simulink model "tx2"  (R2022a)
settings: Solver=FixedStepDiscrete  StartTime=0.0  StopTime=3.1e6  FixedStep=1  RelTol=1e-3
undefined symbols (not defined in the file or in its folder): rom_bf1, rom_bf2, rom_bf3, rom_bf4, rom_bf5, rom_bf6, rom_bf7, rom_bf8, rom_pilot_tt
libraries: hdlsllib x809, whdlutilities x460, whdlmod x104, whdledac x26, simulink x3
(part 25 of 27)

== system tx2/Subsystem4/OFDM_process1/OFDM_process1_bf1/OFDM_BF1/recover_valid_specify ==
  data_in : Inport
  start_in : Inport  Port=2  OutDataTypeStr=boolean
  end_in : Inport  Port=3  OutDataTypeStr=boolean
  Constant : Constant  Value=0  OutDataTypeStr=boolean
  Data Type Conversion1 : DataTypeConversion  OutDataTypeStr=boolean  SaturateOnIntegerOverflow=off  RndMeth=Floor
  Delay : Delay  InitialCondition=0
  Delay1 : Delay  DelayLength=1  InitialCondition=0
  Delay2 : Delay  DelayLength=1  InitialCondition=0
  Delay3 : Delay  InitialCondition=0
  HDL Counter1 : hdlsllib/Sources/HDL Counter  CountType=Count limited  CountInit=0  CountStep=1  CountMax=1  CountFromType=Initial value  CountFrom=0  CountResetPort=off  CountLoadPort=off  CountEnbPort=on  CountDirPort=off  CountHitOutputPort=off  CountDataType=Unsigned  CountWordLen=1  CountFracLen=0  CountSampTime=1
  Logical Operator : Logic  Operator=XOR  AllPortsSameDT=off  OutDataTypeStr=boolean
  Logical Operator1 : Logic  AllPortsSameDT=off  OutDataTypeStr=boolean
  Logical Operator2 : Logic  Operator=NOT  AllPortsSameDT=off  OutDataTypeStr=boolean
  Logical Operator3 : Logic  AllPortsSameDT=off  OutDataTypeStr=boolean
  Logical Operator4 : Logic  AllPortsSameDT=off  OutDataTypeStr=boolean
  Switch : Switch  Criteria=u2 ~= 0  SaturateOnIntegerOverflow=off  InputSameDT=off
  data_out : Outport  VectorParamsAs1DForOutWhenUnconnected=off
  start_out : Outport  Port=2  OutDataTypeStr=boolean  VectorParamsAs1DForOutWhenUnconnected=off
  end_out : Outport  Port=3  OutDataTypeStr=boolean  VectorParamsAs1DForOutWhenUnconnected=off
  valid_out : Outport  Port=4  OutDataTypeStr=boolean  VectorParamsAs1DForOutWhenUnconnected=off
  wires:
  Delay/1 -> Logical Operator/1, Logical Operator1/1, Logical Operator3/1
  Delay3/1 -> data_out/1  "data_out"
  Delay2/1 -> Logical Operator4/2
  Logical Operator/1 -> Switch/3
  Delay1/1 -> Logical Operator/2, Delay2/1  "start_out"
  data_in/1 -> Delay3/1  "data_in"
  end_in/1 -> Delay/1
  Data Type Conversion1/1 -> valid_out/1, Logical Operator3/2, Logical Operator4/1, Logical Operator2/1  "valid_out2"
  HDL Counter1/1 -> Data Type Conversion1/1
  Logical Operator2/1 -> Logical Operator1/2
  Switch/1 -> HDL Counter1/1
  Logical Operator1/1 -> Switch/2
  Constant/1 -> Switch/1
  start_in/1 -> Delay1/1
  Logical Operator4/1 -> start_out/1  "start_out"
  Logical Operator3/1 -> end_out/1  "end_out"

== system tx2/Subsystem4/OFDM_process1/OFDM_process1_bf2/OFDM_BF1/recover_valid_specify ==
  data_in : Inport
  start_in : Inport  Port=2  OutDataTypeStr=boolean
  end_in : Inport  Port=3  OutDataTypeStr=boolean
  Constant : Constant  Value=0  OutDataTypeStr=boolean
  Data Type Conversion1 : DataTypeConversion  OutDataTypeStr=boolean  SaturateOnIntegerOverflow=off  RndMeth=Floor
  Delay : Delay  InitialCondition=0
  Delay1 : Delay  DelayLength=1  InitialCondition=0
  Delay2 : Delay  DelayLength=1  InitialCondition=0
  Delay3 : Delay  InitialCondition=0
  HDL Counter1 : hdlsllib/Sources/HDL Counter  CountType=Count limited  CountInit=0  CountStep=1  CountMax=1  CountFromType=Initial value  CountFrom=0  CountResetPort=off  CountLoadPort=off  CountEnbPort=on  CountDirPort=off  CountHitOutputPort=off  CountDataType=Unsigned  CountWordLen=1  CountFracLen=0  CountSampTime=1
  Logical Operator : Logic  Operator=XOR  AllPortsSameDT=off  OutDataTypeStr=boolean
  Logical Operator1 : Logic  AllPortsSameDT=off  OutDataTypeStr=boolean
  Logical Operator2 : Logic  Operator=NOT  AllPortsSameDT=off  OutDataTypeStr=boolean
  Logical Operator3 : Logic  AllPortsSameDT=off  OutDataTypeStr=boolean
  Logical Operator4 : Logic  AllPortsSameDT=off  OutDataTypeStr=boolean
  Switch : Switch  Criteria=u2 ~= 0  SaturateOnIntegerOverflow=off  InputSameDT=off
  data_out : Outport  VectorParamsAs1DForOutWhenUnconnected=off
  start_out : Outport  Port=2  OutDataTypeStr=boolean  VectorParamsAs1DForOutWhenUnconnected=off
  end_out : Outport  Port=3  OutDataTypeStr=boolean  VectorParamsAs1DForOutWhenUnconnected=off
  valid_out : Outport  Port=4  OutDataTypeStr=boolean  VectorParamsAs1DForOutWhenUnconnected=off
  wires:
  Logical Operator3/1 -> end_out/1  "end_out"
  Logical Operator4/1 -> start_out/1  "start_out"
  start_in/1 -> Delay1/1
  Constant/1 -> Switch/1
  Logical Operator1/1 -> Switch/2
  Switch/1 -> HDL Counter1/1
  Logical Operator2/1 -> Logical Operator1/2
  HDL Counter1/1 -> Data Type Conversion1/1
  Data Type Conversion1/1 -> Logical Operator2/1, Logical Operator4/1, Logical Operator3/2, valid_out/1  "valid_out2"
  end_in/1 -> Delay/1
  data_in/1 -> Delay3/1  "data_in"
  Delay1/1 -> Delay2/1, Logical Operator/2  "start_out"
  Logical Operator/1 -> Switch/3
  Delay2/1 -> Logical Operator4/2
  Delay3/1 -> data_out/1  "data_out"
  Delay/1 -> Logical Operator3/1, Logical Operator1/1, Logical Operator/1

== system tx2/Subsystem4/OFDM_process1/OFDM_process1_bf3/OFDM_BF1/recover_valid_specify ==
  data_in : Inport
  start_in : Inport  Port=2  OutDataTypeStr=boolean
  end_in : Inport  Port=3  OutDataTypeStr=boolean
  Constant : Constant  Value=0  OutDataTypeStr=boolean
  Data Type Conversion1 : DataTypeConversion  OutDataTypeStr=boolean  SaturateOnIntegerOverflow=off  RndMeth=Floor
  Delay : Delay  InitialCondition=0
  Delay1 : Delay  DelayLength=1  InitialCondition=0
  Delay2 : Delay  DelayLength=1  InitialCondition=0
  Delay3 : Delay  InitialCondition=0
  HDL Counter1 : hdlsllib/Sources/HDL Counter  CountType=Count limited  CountInit=0  CountStep=1  CountMax=1  CountFromType=Initial value  CountFrom=0  CountResetPort=off  CountLoadPort=off  CountEnbPort=on  CountDirPort=off  CountHitOutputPort=off  CountDataType=Unsigned  CountWordLen=1  CountFracLen=0  CountSampTime=1
  Logical Operator : Logic  Operator=XOR  AllPortsSameDT=off  OutDataTypeStr=boolean
  Logical Operator1 : Logic  AllPortsSameDT=off  OutDataTypeStr=boolean
  Logical Operator2 : Logic  Operator=NOT  AllPortsSameDT=off  OutDataTypeStr=boolean
  Logical Operator3 : Logic  AllPortsSameDT=off  OutDataTypeStr=boolean
  Logical Operator4 : Logic  AllPortsSameDT=off  OutDataTypeStr=boolean
  Switch : Switch  Criteria=u2 ~= 0  SaturateOnIntegerOverflow=off  InputSameDT=off
  data_out : Outport  VectorParamsAs1DForOutWhenUnconnected=off
  start_out : Outport  Port=2  OutDataTypeStr=boolean  VectorParamsAs1DForOutWhenUnconnected=off
  end_out : Outport  Port=3  OutDataTypeStr=boolean  VectorParamsAs1DForOutWhenUnconnected=off
  valid_out : Outport  Port=4  OutDataTypeStr=boolean  VectorParamsAs1DForOutWhenUnconnected=off
  wires:
  Delay/1 -> Logical Operator/1, Logical Operator1/1, Logical Operator3/1
  Delay3/1 -> data_out/1  "data_out"
  Delay2/1 -> Logical Operator4/2
  Logical Operator/1 -> Switch/3
  Delay1/1 -> Logical Operator/2, Delay2/1  "start_out"
  data_in/1 -> Delay3/1  "data_in"
  end_in/1 -> Delay/1
  Data Type Conversion1/1 -> valid_out/1, Logical Operator3/2, Logical Operator4/1, Logical Operator2/1  "valid_out2"
  HDL Counter1/1 -> Data Type Conversion1/1
  Logical Operator2/1 -> Logical Operator1/2
  Switch/1 -> HDL Counter1/1
  Logical Operator1/1 -> Switch/2
  Constant/1 -> Switch/1
  start_in/1 -> Delay1/1
  Logical Operator4/1 -> start_out/1  "start_out"
  Logical Operator3/1 -> end_out/1  "end_out"

== system tx2/Subsystem4/OFDM_process1/OFDM_process1_bf4/OFDM_BF1/recover_valid_specify ==
  data_in : Inport
  start_in : Inport  Port=2  OutDataTypeStr=boolean
  end_in : Inport  Port=3  OutDataTypeStr=boolean
  Constant : Constant  Value=0  OutDataTypeStr=boolean
  Data Type Conversion1 : DataTypeConversion  OutDataTypeStr=boolean  SaturateOnIntegerOverflow=off  RndMeth=Floor
  Delay : Delay  InitialCondition=0
  Delay1 : Delay  DelayLength=1  InitialCondition=0
  Delay2 : Delay  DelayLength=1  InitialCondition=0
  Delay3 : Delay  InitialCondition=0
  HDL Counter1 : hdlsllib/Sources/HDL Counter  CountType=Count limited  CountInit=0  CountStep=1  CountMax=1  CountFromType=Initial value  CountFrom=0  CountResetPort=off  CountLoadPort=off  CountEnbPort=on  CountDirPort=off  CountHitOutputPort=off  CountDataType=Unsigned  CountWordLen=1  CountFracLen=0  CountSampTime=1
  Logical Operator : Logic  Operator=XOR  AllPortsSameDT=off  OutDataTypeStr=boolean
  Logical Operator1 : Logic  AllPortsSameDT=off  OutDataTypeStr=boolean
  Logical Operator2 : Logic  Operator=NOT  AllPortsSameDT=off  OutDataTypeStr=boolean
  Logical Operator3 : Logic  AllPortsSameDT=off  OutDataTypeStr=boolean
  Logical Operator4 : Logic  AllPortsSameDT=off  OutDataTypeStr=boolean
  Switch : Switch  Criteria=u2 ~= 0  SaturateOnIntegerOverflow=off  InputSameDT=off
  data_out : Outport  VectorParamsAs1DForOutWhenUnconnected=off
  start_out : Outport  Port=2  OutDataTypeStr=boolean  VectorParamsAs1DForOutWhenUnconnected=off
  end_out : Outport  Port=3  OutDataTypeStr=boolean  VectorParamsAs1DForOutWhenUnconnected=off
  valid_out : Outport  Port=4  OutDataTypeStr=boolean  VectorParamsAs1DForOutWhenUnconnected=off
  wires:
  Logical Operator3/1 -> end_out/1  "end_out"
  Logical Operator4/1 -> start_out/1  "start_out"
  start_in/1 -> Delay1/1
  Constant/1 -> Switch/1
  Logical Operator1/1 -> Switch/2
  Switch/1 -> HDL Counter1/1
  Logical Operator2/1 -> Logical Operator1/2
  HDL Counter1/1 -> Data Type Conversion1/1
  Data Type Conversion1/1 -> Logical Operator2/1, Logical Operator4/1, Logical Operator3/2, valid_out/1  "valid_out2"
  end_in/1 -> Delay/1
  data_in/1 -> Delay3/1  "data_in"
  Delay1/1 -> Delay2/1, Logical Operator/2  "start_out"
  Logical Operator/1 -> Switch/3
  Delay2/1 -> Logical Operator4/2
  Delay3/1 -> data_out/1  "data_out"
  Delay/1 -> Logical Operator3/1, Logical Operator1/1, Logical Operator/1

== system tx2/Subsystem4/OFDM_process1/OFDM_process1_bf5/OFDM_BF1/recover_valid_specify ==
  data_in : Inport
  start_in : Inport  Port=2  OutDataTypeStr=boolean
  end_in : Inport  Port=3  OutDataTypeStr=boolean
  Constant : Constant  Value=0  OutDataTypeStr=boolean
  Data Type Conversion1 : DataTypeConversion  OutDataTypeStr=boolean  SaturateOnIntegerOverflow=off  RndMeth=Floor
  Delay : Delay  InitialCondition=0
  Delay1 : Delay  DelayLength=1  InitialCondition=0
  Delay2 : Delay  DelayLength=1  InitialCondition=0
  Delay3 : Delay  InitialCondition=0
  HDL Counter1 : hdlsllib/Sources/HDL Counter  CountType=Count limited  CountInit=0  CountStep=1  CountMax=1  CountFromType=Initial value  CountFrom=0  CountResetPort=off  CountLoadPort=off  CountEnbPort=on  CountDirPort=off  CountHitOutputPort=off  CountDataType=Unsigned  CountWordLen=1  CountFracLen=0  CountSampTime=1
  Logical Operator : Logic  Operator=XOR  AllPortsSameDT=off  OutDataTypeStr=boolean
  Logical Operator1 : Logic  AllPortsSameDT=off  OutDataTypeStr=boolean
  Logical Operator2 : Logic  Operator=NOT  AllPortsSameDT=off  OutDataTypeStr=boolean
  Logical Operator3 : Logic  AllPortsSameDT=off  OutDataTypeStr=boolean
  Logical Operator4 : Logic  AllPortsSameDT=off  OutDataTypeStr=boolean
  Switch : Switch  Criteria=u2 ~= 0  SaturateOnIntegerOverflow=off  InputSameDT=off
  data_out : Outport  VectorParamsAs1DForOutWhenUnconnected=off
  start_out : Outport  Port=2  OutDataTypeStr=boolean  VectorParamsAs1DForOutWhenUnconnected=off
  end_out : Outport  Port=3  OutDataTypeStr=boolean  VectorParamsAs1DForOutWhenUnconnected=off
  valid_out : Outport  Port=4  OutDataTypeStr=boolean  VectorParamsAs1DForOutWhenUnconnected=off
  wires:
  Delay/1 -> Logical Operator/1, Logical Operator1/1, Logical Operator3/1
  Delay3/1 -> data_out/1  "data_out"
  Delay2/1 -> Logical Operator4/2
  Logical Operator/1 -> Switch/3
  Delay1/1 -> Logical Operator/2, Delay2/1  "start_out"
  data_in/1 -> Delay3/1  "data_in"
  end_in/1 -> Delay/1
  Data Type Conversion1/1 -> valid_out/1, Logical Operator3/2, Logical Operator4/1, Logical Operator2/1  "valid_out2"
  HDL Counter1/1 -> Data Type Conversion1/1
  Logical Operator2/1 -> Logical Operator1/2
  Switch/1 -> HDL Counter1/1
  Logical Operator1/1 -> Switch/2
  Constant/1 -> Switch/1
  start_in/1 -> Delay1/1
  Logical Operator4/1 -> start_out/1  "start_out"
  Logical Operator3/1 -> end_out/1  "end_out"

== system tx2/Subsystem4/OFDM_process1/OFDM_process1_bf6/OFDM_BF1/recover_valid_specify ==
  data_in : Inport
  start_in : Inport  Port=2  OutDataTypeStr=boolean
  end_in : Inport  Port=3  OutDataTypeStr=boolean
  Constant : Constant  Value=0  OutDataTypeStr=boolean
  Data Type Conversion1 : DataTypeConversion  OutDataTypeStr=boolean  SaturateOnIntegerOverflow=off  RndMeth=Floor
  Delay : Delay  InitialCondition=0
  Delay1 : Delay  DelayLength=1  InitialCondition=0
  Delay2 : Delay  DelayLength=1  InitialCondition=0
  Delay3 : Delay  InitialCondition=0
  HDL Counter1 : hdlsllib/Sources/HDL Counter  CountType=Count limited  CountInit=0  CountStep=1  CountMax=1  CountFromType=Initial value  CountFrom=0  CountResetPort=off  CountLoadPort=off  CountEnbPort=on  CountDirPort=off  CountHitOutputPort=off  CountDataType=Unsigned  CountWordLen=1  CountFracLen=0  CountSampTime=1
  Logical Operator : Logic  Operator=XOR  AllPortsSameDT=off  OutDataTypeStr=boolean
  Logical Operator1 : Logic  AllPortsSameDT=off  OutDataTypeStr=boolean
  Logical Operator2 : Logic  Operator=NOT  AllPortsSameDT=off  OutDataTypeStr=boolean
  Logical Operator3 : Logic  AllPortsSameDT=off  OutDataTypeStr=boolean
  Logical Operator4 : Logic  AllPortsSameDT=off  OutDataTypeStr=boolean
  Switch : Switch  Criteria=u2 ~= 0  SaturateOnIntegerOverflow=off  InputSameDT=off
  data_out : Outport  VectorParamsAs1DForOutWhenUnconnected=off
  start_out : Outport  Port=2  OutDataTypeStr=boolean  VectorParamsAs1DForOutWhenUnconnected=off
  end_out : Outport  Port=3  OutDataTypeStr=boolean  VectorParamsAs1DForOutWhenUnconnected=off
  valid_out : Outport  Port=4  OutDataTypeStr=boolean  VectorParamsAs1DForOutWhenUnconnected=off
  wires:
  Logical Operator3/1 -> end_out/1  "end_out"
  Logical Operator4/1 -> start_out/1  "start_out"
  start_in/1 -> Delay1/1
  Constant/1 -> Switch/1
  Logical Operator1/1 -> Switch/2
  Switch/1 -> HDL Counter1/1
  Logical Operator2/1 -> Logical Operator1/2
  HDL Counter1/1 -> Data Type Conversion1/1
  Data Type Conversion1/1 -> Logical Operator2/1, Logical Operator4/1, Logical Operator3/2, valid_out/1  "valid_out2"
  end_in/1 -> Delay/1
  data_in/1 -> Delay3/1  "data_in"
  Delay1/1 -> Delay2/1, Logical Operator/2  "start_out"
  Logical Operator/1 -> Switch/3
  Delay2/1 -> Logical Operator4/2
  Delay3/1 -> data_out/1  "data_out"
  Delay/1 -> Logical Operator3/1, Logical Operator1/1, Logical Operator/1

== system tx2/Subsystem4/OFDM_process1/OFDM_process1_bf7/OFDM_BF1/recover_valid_specify ==
  data_in : Inport
  start_in : Inport  Port=2  OutDataTypeStr=boolean
  end_in : Inport  Port=3  OutDataTypeStr=boolean
  Constant : Constant  Value=0  OutDataTypeStr=boolean
  Data Type Conversion1 : DataTypeConversion  OutDataTypeStr=boolean  SaturateOnIntegerOverflow=off  RndMeth=Floor
  Delay : Delay  InitialCondition=0
  Delay1 : Delay  DelayLength=1  InitialCondition=0
  Delay2 : Delay  DelayLength=1  InitialCondition=0
  Delay3 : Delay  InitialCondition=0
  HDL Counter1 : hdlsllib/Sources/HDL Counter  CountType=Count limited  CountInit=0  CountStep=1  CountMax=1  CountFromType=Initial value  CountFrom=0  CountResetPort=off  CountLoadPort=off  CountEnbPort=on  CountDirPort=off  CountHitOutputPort=off  CountDataType=Unsigned  CountWordLen=1  CountFracLen=0  CountSampTime=1
  Logical Operator : Logic  Operator=XOR  AllPortsSameDT=off  OutDataTypeStr=boolean
  Logical Operator1 : Logic  AllPortsSameDT=off  OutDataTypeStr=boolean
  Logical Operator2 : Logic  Operator=NOT  AllPortsSameDT=off  OutDataTypeStr=boolean
  Logical Operator3 : Logic  AllPortsSameDT=off  OutDataTypeStr=boolean
  Logical Operator4 : Logic  AllPortsSameDT=off  OutDataTypeStr=boolean
  Switch : Switch  Criteria=u2 ~= 0  SaturateOnIntegerOverflow=off  InputSameDT=off
  data_out : Outport  VectorParamsAs1DForOutWhenUnconnected=off
  start_out : Outport  Port=2  OutDataTypeStr=boolean  VectorParamsAs1DForOutWhenUnconnected=off
  end_out : Outport  Port=3  OutDataTypeStr=boolean  VectorParamsAs1DForOutWhenUnconnected=off
  valid_out : Outport  Port=4  OutDataTypeStr=boolean  VectorParamsAs1DForOutWhenUnconnected=off
  wires:
  Delay/1 -> Logical Operator/1, Logical Operator1/1, Logical Operator3/1
  Delay3/1 -> data_out/1  "data_out"
  Delay2/1 -> Logical Operator4/2
  Logical Operator/1 -> Switch/3
  Delay1/1 -> Logical Operator/2, Delay2/1  "start_out"
  data_in/1 -> Delay3/1  "data_in"
  end_in/1 -> Delay/1
  Data Type Conversion1/1 -> valid_out/1, Logical Operator3/2, Logical Operator4/1, Logical Operator2/1  "valid_out2"
  HDL Counter1/1 -> Data Type Conversion1/1
  Logical Operator2/1 -> Logical Operator1/2
  Switch/1 -> HDL Counter1/1
  Logical Operator1/1 -> Switch/2
  Constant/1 -> Switch/1
  start_in/1 -> Delay1/1
  Logical Operator4/1 -> start_out/1  "start_out"
  Logical Operator3/1 -> end_out/1  "end_out"

== system tx2/Subsystem4/OFDM_process1/OFDM_process1_bf8/OFDM_BF1/recover_valid_specify ==
  data_in : Inport
  start_in : Inport  Port=2  OutDataTypeStr=boolean
  end_in : Inport  Port=3  OutDataTypeStr=boolean
  Constant : Constant  Value=0  OutDataTypeStr=boolean
  Data Type Conversion1 : DataTypeConversion  OutDataTypeStr=boolean  SaturateOnIntegerOverflow=off  RndMeth=Floor
  Delay : Delay  InitialCondition=0
  Delay1 : Delay  DelayLength=1  InitialCondition=0
  Delay2 : Delay  DelayLength=1  InitialCondition=0
  Delay3 : Delay  InitialCondition=0
  HDL Counter1 : hdlsllib/Sources/HDL Counter  CountType=Count limited  CountInit=0  CountStep=1  CountMax=1  CountFromType=Initial value  CountFrom=0  CountResetPort=off  CountLoadPort=off  CountEnbPort=on  CountDirPort=off  CountHitOutputPort=off  CountDataType=Unsigned  CountWordLen=1  CountFracLen=0  CountSampTime=1
  Logical Operator : Logic  Operator=XOR  AllPortsSameDT=off  OutDataTypeStr=boolean
  Logical Operator1 : Logic  AllPortsSameDT=off  OutDataTypeStr=boolean
  Logical Operator2 : Logic  Operator=NOT  AllPortsSameDT=off  OutDataTypeStr=boolean
  Logical Operator3 : Logic  AllPortsSameDT=off  OutDataTypeStr=boolean
  Logical Operator4 : Logic  AllPortsSameDT=off  OutDataTypeStr=boolean
  Switch : Switch  Criteria=u2 ~= 0  SaturateOnIntegerOverflow=off  InputSameDT=off
  data_out : Outport  VectorParamsAs1DForOutWhenUnconnected=off
  start_out : Outport  Port=2  OutDataTypeStr=boolean  VectorParamsAs1DForOutWhenUnconnected=off
  end_out : Outport  Port=3  OutDataTypeStr=boolean  VectorParamsAs1DForOutWhenUnconnected=off
  valid_out : Outport  Port=4  OutDataTypeStr=boolean  VectorParamsAs1DForOutWhenUnconnected=off
  wires:
  Logical Operator3/1 -> end_out/1  "end_out"
  Logical Operator4/1 -> start_out/1  "start_out"
  start_in/1 -> Delay1/1
  Constant/1 -> Switch/1
  Logical Operator1/1 -> Switch/2
  Switch/1 -> HDL Counter1/1
  Logical Operator2/1 -> Logical Operator1/2
  HDL Counter1/1 -> Data Type Conversion1/1
  Data Type Conversion1/1 -> Logical Operator2/1, Logical Operator4/1, Logical Operator3/2, valid_out/1  "valid_out2"
  end_in/1 -> Delay/1
  data_in/1 -> Delay3/1  "data_in"
  Delay1/1 -> Delay2/1, Logical Operator/2  "start_out"
  Logical Operator/1 -> Switch/3
  Delay2/1 -> Logical Operator4/2
  Delay3/1 -> data_out/1  "data_out"
  Delay/1 -> Logical Operator3/1, Logical Operator1/1, Logical Operator/1

== system tx2/Subsystem5/OFDM_process1/OFDM_process1_bf1/OFDM_BF1/recover_valid_specify ==
  data_in : Inport
  start_in : Inport  Port=2  OutDataTypeStr=boolean
  end_in : Inport  Port=3  OutDataTypeStr=boolean
  Constant : Constant  Value=0  OutDataTypeStr=boolean
  Data Type Conversion1 : DataTypeConversion  OutDataTypeStr=boolean  SaturateOnIntegerOverflow=off  RndMeth=Floor
  Delay : Delay  InitialCondition=0
  Delay1 : Delay  DelayLength=1  InitialCondition=0
  Delay2 : Delay  DelayLength=1  InitialCondition=0
  Delay3 : Delay  InitialCondition=0
  HDL Counter1 : hdlsllib/Sources/HDL Counter  CountType=Count limited  CountInit=0  CountStep=1  CountMax=1  CountFromType=Initial value  CountFrom=0  CountResetPort=off  CountLoadPort=off  CountEnbPort=on  CountDirPort=off  CountHitOutputPort=off  CountDataType=Unsigned  CountWordLen=1  CountFracLen=0  CountSampTime=1
  Logical Operator : Logic  Operator=XOR  AllPortsSameDT=off  OutDataTypeStr=boolean
  Logical Operator1 : Logic  AllPortsSameDT=off  OutDataTypeStr=boolean
  Logical Operator2 : Logic  Operator=NOT  AllPortsSameDT=off  OutDataTypeStr=boolean
  Logical Operator3 : Logic  AllPortsSameDT=off  OutDataTypeStr=boolean
  Logical Operator4 : Logic  AllPortsSameDT=off  OutDataTypeStr=boolean
  Switch : Switch  Criteria=u2 ~= 0  SaturateOnIntegerOverflow=off  InputSameDT=off
  data_out : Outport  VectorParamsAs1DForOutWhenUnconnected=off
  start_out : Outport  Port=2  OutDataTypeStr=boolean  VectorParamsAs1DForOutWhenUnconnected=off
  end_out : Outport  Port=3  OutDataTypeStr=boolean  VectorParamsAs1DForOutWhenUnconnected=off
  valid_out : Outport  Port=4  OutDataTypeStr=boolean  VectorParamsAs1DForOutWhenUnconnected=off
  wires:
  Logical Operator3/1 -> end_out/1  "end_out"
  Logical Operator4/1 -> start_out/1  "start_out"
  start_in/1 -> Delay1/1
  Constant/1 -> Switch/1
  Logical Operator1/1 -> Switch/2
  Switch/1 -> HDL Counter1/1
  Logical Operator2/1 -> Logical Operator1/2
  HDL Counter1/1 -> Data Type Conversion1/1
  Data Type Conversion1/1 -> Logical Operator2/1, Logical Operator4/1, Logical Operator3/2, valid_out/1  "valid_out2"
  end_in/1 -> Delay/1
  data_in/1 -> Delay3/1  "data_in"
  Delay1/1 -> Delay2/1, Logical Operator/2  "start_out"
  Logical Operator/1 -> Switch/3
  Delay2/1 -> Logical Operator4/2
  Delay3/1 -> data_out/1  "data_out"
  Delay/1 -> Logical Operator3/1, Logical Operator1/1, Logical Operator/1

== system tx2/Subsystem5/OFDM_process1/OFDM_process1_bf2/OFDM_BF1/recover_valid_specify ==
  data_in : Inport
  start_in : Inport  Port=2  OutDataTypeStr=boolean
  end_in : Inport  Port=3  OutDataTypeStr=boolean
  Constant : Constant  Value=0  OutDataTypeStr=boolean
  Data Type Conversion1 : DataTypeConversion  OutDataTypeStr=boolean  SaturateOnIntegerOverflow=off  RndMeth=Floor
  Delay : Delay  InitialCondition=0
  Delay1 : Delay  DelayLength=1  InitialCondition=0
  Delay2 : Delay  DelayLength=1  InitialCondition=0
  Delay3 : Delay  InitialCondition=0
  HDL Counter1 : hdlsllib/Sources/HDL Counter  CountType=Count limited  CountInit=0  CountStep=1  CountMax=1  CountFromType=Initial value  CountFrom=0  CountResetPort=off  CountLoadPort=off  CountEnbPort=on  CountDirPort=off  CountHitOutputPort=off  CountDataType=Unsigned  CountWordLen=1  CountFracLen=0  CountSampTime=1
  Logical Operator : Logic  Operator=XOR  AllPortsSameDT=off  OutDataTypeStr=boolean
  Logical Operator1 : Logic  AllPortsSameDT=off  OutDataTypeStr=boolean
  Logical Operator2 : Logic  Operator=NOT  AllPortsSameDT=off  OutDataTypeStr=boolean
  Logical Operator3 : Logic  AllPortsSameDT=off  OutDataTypeStr=boolean
  Logical Operator4 : Logic  AllPortsSameDT=off  OutDataTypeStr=boolean
  Switch : Switch  Criteria=u2 ~= 0  SaturateOnIntegerOverflow=off  InputSameDT=off
  data_out : Outport  VectorParamsAs1DForOutWhenUnconnected=off
  start_out : Outport  Port=2  OutDataTypeStr=boolean  VectorParamsAs1DForOutWhenUnconnected=off
  end_out : Outport  Port=3  OutDataTypeStr=boolean  VectorParamsAs1DForOutWhenUnconnected=off
  valid_out : Outport  Port=4  OutDataTypeStr=boolean  VectorParamsAs1DForOutWhenUnconnected=off
  wires:
  Delay/1 -> Logical Operator/1, Logical Operator1/1, Logical Operator3/1
  Delay3/1 -> data_out/1  "data_out"
  Delay2/1 -> Logical Operator4/2
  Logical Operator/1 -> Switch/3
  Delay1/1 -> Logical Operator/2, Delay2/1  "start_out"
  data_in/1 -> Delay3/1  "data_in"
  end_in/1 -> Delay/1
  Data Type Conversion1/1 -> valid_out/1, Logical Operator3/2, Logical Operator4/1, Logical Operator2/1  "valid_out2"
  HDL Counter1/1 -> Data Type Conversion1/1
  Logical Operator2/1 -> Logical Operator1/2
  Switch/1 -> HDL Counter1/1
  Logical Operator1/1 -> Switch/2
  Constant/1 -> Switch/1
  start_in/1 -> Delay1/1
  Logical Operator4/1 -> start_out/1  "start_out"
  Logical Operator3/1 -> end_out/1  "end_out"

== system tx2/Subsystem5/OFDM_process1/OFDM_process1_bf3/OFDM_BF1/recover_valid_specify ==
  data_in : Inport
  start_in : Inport  Port=2  OutDataTypeStr=boolean
  end_in : Inport  Port=3  OutDataTypeStr=boolean
  Constant : Constant  Value=0  OutDataTypeStr=boolean
  Data Type Conversion1 : DataTypeConversion  OutDataTypeStr=boolean  SaturateOnIntegerOverflow=off  RndMeth=Floor
  Delay : Delay  InitialCondition=0
  Delay1 : Delay  DelayLength=1  InitialCondition=0
  Delay2 : Delay  DelayLength=1  InitialCondition=0
  Delay3 : Delay  InitialCondition=0
  HDL Counter1 : hdlsllib/Sources/HDL Counter  CountType=Count limited  CountInit=0  CountStep=1  CountMax=1  CountFromType=Initial value  CountFrom=0  CountResetPort=off  CountLoadPort=off  CountEnbPort=on  CountDirPort=off  CountHitOutputPort=off  CountDataType=Unsigned  CountWordLen=1  CountFracLen=0  CountSampTime=1
  Logical Operator : Logic  Operator=XOR  AllPortsSameDT=off  OutDataTypeStr=boolean
  Logical Operator1 : Logic  AllPortsSameDT=off  OutDataTypeStr=boolean
  Logical Operator2 : Logic  Operator=NOT  AllPortsSameDT=off  OutDataTypeStr=boolean
  Logical Operator3 : Logic  AllPortsSameDT=off  OutDataTypeStr=boolean
  Logical Operator4 : Logic  AllPortsSameDT=off  OutDataTypeStr=boolean
  Switch : Switch  Criteria=u2 ~= 0  SaturateOnIntegerOverflow=off  InputSameDT=off
  data_out : Outport  VectorParamsAs1DForOutWhenUnconnected=off
  start_out : Outport  Port=2  OutDataTypeStr=boolean  VectorParamsAs1DForOutWhenUnconnected=off
  end_out : Outport  Port=3  OutDataTypeStr=boolean  VectorParamsAs1DForOutWhenUnconnected=off
  valid_out : Outport  Port=4  OutDataTypeStr=boolean  VectorParamsAs1DForOutWhenUnconnected=off
  wires:
  Logical Operator3/1 -> end_out/1  "end_out"
  Logical Operator4/1 -> start_out/1  "start_out"
  start_in/1 -> Delay1/1
  Constant/1 -> Switch/1
  Logical Operator1/1 -> Switch/2
  Switch/1 -> HDL Counter1/1
  Logical Operator2/1 -> Logical Operator1/2
  HDL Counter1/1 -> Data Type Conversion1/1
  Data Type Conversion1/1 -> Logical Operator2/1, Logical Operator4/1, Logical Operator3/2, valid_out/1  "valid_out2"
  end_in/1 -> Delay/1
  data_in/1 -> Delay3/1  "data_in"
  Delay1/1 -> Delay2/1, Logical Operator/2  "start_out"
  Logical Operator/1 -> Switch/3
  Delay2/1 -> Logical Operator4/2
  Delay3/1 -> data_out/1  "data_out"
  Delay/1 -> Logical Operator3/1, Logical Operator1/1, Logical Operator/1

== system tx2/Subsystem5/OFDM_process1/OFDM_process1_bf4/OFDM_BF1/recover_valid_specify ==
  data_in : Inport
  start_in : Inport  Port=2  OutDataTypeStr=boolean
  end_in : Inport  Port=3  OutDataTypeStr=boolean
  Constant : Constant  Value=0  OutDataTypeStr=boolean
  Data Type Conversion1 : DataTypeConversion  OutDataTypeStr=boolean  SaturateOnIntegerOverflow=off  RndMeth=Floor
  Delay : Delay  InitialCondition=0
  Delay1 : Delay  DelayLength=1  InitialCondition=0
  Delay2 : Delay  DelayLength=1  InitialCondition=0
  Delay3 : Delay  InitialCondition=0
  HDL Counter1 : hdlsllib/Sources/HDL Counter  CountType=Count limited  CountInit=0  CountStep=1  CountMax=1  CountFromType=Initial value  CountFrom=0  CountResetPort=off  CountLoadPort=off  CountEnbPort=on  CountDirPort=off  CountHitOutputPort=off  CountDataType=Unsigned  CountWordLen=1  CountFracLen=0  CountSampTime=1
  Logical Operator : Logic  Operator=XOR  AllPortsSameDT=off  OutDataTypeStr=boolean
  Logical Operator1 : Logic  AllPortsSameDT=off  OutDataTypeStr=boolean
  Logical Operator2 : Logic  Operator=NOT  AllPortsSameDT=off  OutDataTypeStr=boolean
  Logical Operator3 : Logic  AllPortsSameDT=off  OutDataTypeStr=boolean
  Logical Operator4 : Logic  AllPortsSameDT=off  OutDataTypeStr=boolean
  Switch : Switch  Criteria=u2 ~= 0  SaturateOnIntegerOverflow=off  InputSameDT=off
  data_out : Outport  VectorParamsAs1DForOutWhenUnconnected=off
  start_out : Outport  Port=2  OutDataTypeStr=boolean  VectorParamsAs1DForOutWhenUnconnected=off
  end_out : Outport  Port=3  OutDataTypeStr=boolean  VectorParamsAs1DForOutWhenUnconnected=off
  valid_out : Outport  Port=4  OutDataTypeStr=boolean  VectorParamsAs1DForOutWhenUnconnected=off
  wires:
  Delay/1 -> Logical Operator/1, Logical Operator1/1, Logical Operator3/1
  Delay3/1 -> data_out/1  "data_out"
  Delay2/1 -> Logical Operator4/2
  Logical Operator/1 -> Switch/3
  Delay1/1 -> Logical Operator/2, Delay2/1  "start_out"
  data_in/1 -> Delay3/1  "data_in"
  end_in/1 -> Delay/1
  Data Type Conversion1/1 -> valid_out/1, Logical Operator3/2, Logical Operator4/1, Logical Operator2/1  "valid_out2"
  HDL Counter1/1 -> Data Type Conversion1/1
  Logical Operator2/1 -> Logical Operator1/2
  Switch/1 -> HDL Counter1/1
  Logical Operator1/1 -> Switch/2
  Constant/1 -> Switch/1
  start_in/1 -> Delay1/1
  Logical Operator4/1 -> start_out/1  "start_out"
  Logical Operator3/1 -> end_out/1  "end_out"

== system tx2/Subsystem5/OFDM_process1/OFDM_process1_bf5/OFDM_BF1/recover_valid_specify ==
  data_in : Inport
  start_in : Inport  Port=2  OutDataTypeStr=boolean
  end_in : Inport  Port=3  OutDataTypeStr=boolean
  Constant : Constant  Value=0  OutDataTypeStr=boolean
  Data Type Conversion1 : DataTypeConversion  OutDataTypeStr=boolean  SaturateOnIntegerOverflow=off  RndMeth=Floor
  Delay : Delay  InitialCondition=0
  Delay1 : Delay  DelayLength=1  InitialCondition=0
  Delay2 : Delay  DelayLength=1  InitialCondition=0
  Delay3 : Delay  InitialCondition=0
  HDL Counter1 : hdlsllib/Sources/HDL Counter  CountType=Count limited  CountInit=0  CountStep=1  CountMax=1  CountFromType=Initial value  CountFrom=0  CountResetPort=off  CountLoadPort=off  CountEnbPort=on  CountDirPort=off  CountHitOutputPort=off  CountDataType=Unsigned  CountWordLen=1  CountFracLen=0  CountSampTime=1
  Logical Operator : Logic  Operator=XOR  AllPortsSameDT=off  OutDataTypeStr=boolean
  Logical Operator1 : Logic  AllPortsSameDT=off  OutDataTypeStr=boolean
  Logical Operator2 : Logic  Operator=NOT  AllPortsSameDT=off  OutDataTypeStr=boolean
  Logical Operator3 : Logic  AllPortsSameDT=off  OutDataTypeStr=boolean
  Logical Operator4 : Logic  AllPortsSameDT=off  OutDataTypeStr=boolean
  Switch : Switch  Criteria=u2 ~= 0  SaturateOnIntegerOverflow=off  InputSameDT=off
  data_out : Outport  VectorParamsAs1DForOutWhenUnconnected=off
  start_out : Outport  Port=2  OutDataTypeStr=boolean  VectorParamsAs1DForOutWhenUnconnected=off
  end_out : Outport  Port=3  OutDataTypeStr=boolean  VectorParamsAs1DForOutWhenUnconnected=off
  valid_out : Outport  Port=4  OutDataTypeStr=boolean  VectorParamsAs1DForOutWhenUnconnected=off
  wires:
  Logical Operator3/1 -> end_out/1  "end_out"
  Logical Operator4/1 -> start_out/1  "start_out"
  start_in/1 -> Delay1/1
  Constant/1 -> Switch/1
  Logical Operator1/1 -> Switch/2
  Switch/1 -> HDL Counter1/1
  Logical Operator2/1 -> Logical Operator1/2
  HDL Counter1/1 -> Data Type Conversion1/1
  Data Type Conversion1/1 -> Logical Operator2/1, Logical Operator4/1, Logical Operator3/2, valid_out/1  "valid_out2"
  end_in/1 -> Delay/1
  data_in/1 -> Delay3/1  "data_in"
  Delay1/1 -> Delay2/1, Logical Operator/2  "start_out"
  Logical Operator/1 -> Switch/3
  Delay2/1 -> Logical Operator4/2
  Delay3/1 -> data_out/1  "data_out"
  Delay/1 -> Logical Operator3/1, Logical Operator1/1, Logical Operator/1

== system tx2/Subsystem5/OFDM_process1/OFDM_process1_bf6/OFDM_BF1/recover_valid_specify ==
  data_in : Inport
  start_in : Inport  Port=2  OutDataTypeStr=boolean
  end_in : Inport  Port=3  OutDataTypeStr=boolean
  Constant : Constant  Value=0  OutDataTypeStr=boolean
  Data Type Conversion1 : DataTypeConversion  OutDataTypeStr=boolean  SaturateOnIntegerOverflow=off  RndMeth=Floor
  Delay : Delay  InitialCondition=0
  Delay1 : Delay  DelayLength=1  InitialCondition=0
  Delay2 : Delay  DelayLength=1  InitialCondition=0
  Delay3 : Delay  InitialCondition=0
  HDL Counter1 : hdlsllib/Sources/HDL Counter  CountType=Count limited  CountInit=0  CountStep=1  CountMax=1  CountFromType=Initial value  CountFrom=0  CountResetPort=off  CountLoadPort=off  CountEnbPort=on  CountDirPort=off  CountHitOutputPort=off  CountDataType=Unsigned  CountWordLen=1  CountFracLen=0  CountSampTime=1
  Logical Operator : Logic  Operator=XOR  AllPortsSameDT=off  OutDataTypeStr=boolean
  Logical Operator1 : Logic  AllPortsSameDT=off  OutDataTypeStr=boolean
  Logical Operator2 : Logic  Operator=NOT  AllPortsSameDT=off  OutDataTypeStr=boolean
  Logical Operator3 : Logic  AllPortsSameDT=off  OutDataTypeStr=boolean
  Logical Operator4 : Logic  AllPortsSameDT=off  OutDataTypeStr=boolean
  Switch : Switch  Criteria=u2 ~= 0  SaturateOnIntegerOverflow=off  InputSameDT=off
  data_out : Outport  VectorParamsAs1DForOutWhenUnconnected=off
  start_out : Outport  Port=2  OutDataTypeStr=boolean  VectorParamsAs1DForOutWhenUnconnected=off
  end_out : Outport  Port=3  OutDataTypeStr=boolean  VectorParamsAs1DForOutWhenUnconnected=off
  valid_out : Outport  Port=4  OutDataTypeStr=boolean  VectorParamsAs1DForOutWhenUnconnected=off
  wires:
  Delay/1 -> Logical Operator/1, Logical Operator1/1, Logical Operator3/1
  Delay3/1 -> data_out/1  "data_out"
  Delay2/1 -> Logical Operator4/2
  Logical Operator/1 -> Switch/3
  Delay1/1 -> Logical Operator/2, Delay2/1  "start_out"
  data_in/1 -> Delay3/1  "data_in"
  end_in/1 -> Delay/1
  Data Type Conversion1/1 -> valid_out/1, Logical Operator3/2, Logical Operator4/1, Logical Operator2/1  "valid_out2"
  HDL Counter1/1 -> Data Type Conversion1/1
  Logical Operator2/1 -> Logical Operator1/2
  Switch/1 -> HDL Counter1/1
  Logical Operator1/1 -> Switch/2
  Constant/1 -> Switch/1
  start_in/1 -> Delay1/1
  Logical Operator4/1 -> start_out/1  "start_out"
  Logical Operator3/1 -> end_out/1  "end_out"

== system tx2/Subsystem5/OFDM_process1/OFDM_process1_bf7/OFDM_BF1/recover_valid_specify ==
  data_in : Inport
  start_in : Inport  Port=2  OutDataTypeStr=boolean
  end_in : Inport  Port=3  OutDataTypeStr=boolean
  Constant : Constant  Value=0  OutDataTypeStr=boolean
  Data Type Conversion1 : DataTypeConversion  OutDataTypeStr=boolean  SaturateOnIntegerOverflow=off  RndMeth=Floor
  Delay : Delay  InitialCondition=0
  Delay1 : Delay  DelayLength=1  InitialCondition=0
  Delay2 : Delay  DelayLength=1  InitialCondition=0
  Delay3 : Delay  InitialCondition=0
  HDL Counter1 : hdlsllib/Sources/HDL Counter  CountType=Count limited  CountInit=0  CountStep=1  CountMax=1  CountFromType=Initial value  CountFrom=0  CountResetPort=off  CountLoadPort=off  CountEnbPort=on  CountDirPort=off  CountHitOutputPort=off  CountDataType=Unsigned  CountWordLen=1  CountFracLen=0  CountSampTime=1
  Logical Operator : Logic  Operator=XOR  AllPortsSameDT=off  OutDataTypeStr=boolean
  Logical Operator1 : Logic  AllPortsSameDT=off  OutDataTypeStr=boolean
  Logical Operator2 : Logic  Operator=NOT  AllPortsSameDT=off  OutDataTypeStr=boolean
  Logical Operator3 : Logic  AllPortsSameDT=off  OutDataTypeStr=boolean
  Logical Operator4 : Logic  AllPortsSameDT=off  OutDataTypeStr=boolean
  Switch : Switch  Criteria=u2 ~= 0  SaturateOnIntegerOverflow=off  InputSameDT=off
  data_out : Outport  VectorParamsAs1DForOutWhenUnconnected=off
  start_out : Outport  Port=2  OutDataTypeStr=boolean  VectorParamsAs1DForOutWhenUnconnected=off
  end_out : Outport  Port=3  OutDataTypeStr=boolean  VectorParamsAs1DForOutWhenUnconnected=off
  valid_out : Outport  Port=4  OutDataTypeStr=boolean  VectorParamsAs1DForOutWhenUnconnected=off
  wires:
  Logical Operator3/1 -> end_out/1  "end_out"
  Logical Operator4/1 -> start_out/1  "start_out"
  start_in/1 -> Delay1/1
  Constant/1 -> Switch/1
  Logical Operator1/1 -> Switch/2
  Switch/1 -> HDL Counter1/1
  Logical Operator2/1 -> Logical Operator1/2
  HDL Counter1/1 -> Data Type Conversion1/1
  Data Type Conversion1/1 -> Logical Operator2/1, Logical Operator4/1, Logical Operator3/2, valid_out/1  "valid_out2"
  end_in/1 -> Delay/1
  data_in/1 -> Delay3/1  "data_in"
  Delay1/1 -> Delay2/1, Logical Operator/2  "start_out"
  Logical Operator/1 -> Switch/3
  Delay2/1 -> Logical Operator4/2
  Delay3/1 -> data_out/1  "data_out"
  Delay/1 -> Logical Operator3/1, Logical Operator1/1, Logical Operator/1

== system tx2/Subsystem5/OFDM_process1/OFDM_process1_bf8/OFDM_BF1/recover_valid_specify ==
  data_in : Inport
  start_in : Inport  Port=2  OutDataTypeStr=boolean
  end_in : Inport  Port=3  OutDataTypeStr=boolean
  Constant : Constant  Value=0  OutDataTypeStr=boolean
  Data Type Conversion1 : DataTypeConversion  OutDataTypeStr=boolean  SaturateOnIntegerOverflow=off  RndMeth=Floor
  Delay : Delay  InitialCondition=0
  Delay1 : Delay  DelayLength=1  InitialCondition=0
  Delay2 : Delay  DelayLength=1  InitialCondition=0
  Delay3 : Delay  InitialCondition=0
  HDL Counter1 : hdlsllib/Sources/HDL Counter  CountType=Count limited  CountInit=0  CountStep=1  CountMax=1  CountFromType=Initial value  CountFrom=0  CountResetPort=off  CountLoadPort=off  CountEnbPort=on  CountDirPort=off  CountHitOutputPort=off  CountDataType=Unsigned  CountWordLen=1  CountFracLen=0  CountSampTime=1
  Logical Operator : Logic  Operator=XOR  AllPortsSameDT=off  OutDataTypeStr=boolean
  Logical Operator1 : Logic  AllPortsSameDT=off  OutDataTypeStr=boolean
  Logical Operator2 : Logic  Operator=NOT  AllPortsSameDT=off  OutDataTypeStr=boolean
  Logical Operator3 : Logic  AllPortsSameDT=off  OutDataTypeStr=boolean
  Logical Operator4 : Logic  AllPortsSameDT=off  OutDataTypeStr=boolean
  Switch : Switch  Criteria=u2 ~= 0  SaturateOnIntegerOverflow=off  InputSameDT=off
  data_out : Outport  VectorParamsAs1DForOutWhenUnconnected=off
  start_out : Outport  Port=2  OutDataTypeStr=boolean  VectorParamsAs1DForOutWhenUnconnected=off
  end_out : Outport  Port=3  OutDataTypeStr=boolean  VectorParamsAs1DForOutWhenUnconnected=off
  valid_out : Outport  Port=4  OutDataTypeStr=boolean  VectorParamsAs1DForOutWhenUnconnected=off
  wires:
  Delay/1 -> Logical Operator/1, Logical Operator1/1, Logical Operator3/1
  Delay3/1 -> data_out/1  "data_out"
  Delay2/1 -> Logical Operator4/2
  Logical Operator/1 -> Switch/3
  Delay1/1 -> Logical Operator/2, Delay2/1  "start_out"
  data_in/1 -> Delay3/1  "data_in"
  end_in/1 -> Delay/1
  Data Type Conversion1/1 -> valid_out/1, Logical Operator3/2, Logical Operator4/1, Logical Operator2/1  "valid_out2"
  HDL Counter1/1 -> Data Type Conversion1/1
  Logical Operator2/1 -> Logical Operator1/2
  Switch/1 -> HDL Counter1/1
  Logical Operator1/1 -> Switch/2
  Constant/1 -> Switch/1
  start_in/1 -> Delay1/1
  Logical Operator4/1 -> start_out/1  "start_out"
  Logical Operator3/1 -> end_out/1  "end_out"

== system tx2/Subsystem6/OFDM_process1/OFDM_process1_bf1/OFDM_BF1/recover_valid_specify ==
  data_in : Inport
  start_in : Inport  Port=2  OutDataTypeStr=boolean
  end_in : Inport  Port=3  OutDataTypeStr=boolean
  Constant : Constant  Value=0  OutDataTypeStr=boolean
  Data Type Conversion1 : DataTypeConversion  OutDataTypeStr=boolean  SaturateOnIntegerOverflow=off  RndMeth=Floor
  Delay : Delay  InitialCondition=0
  Delay1 : Delay  DelayLength=1  InitialCondition=0
  Delay2 : Delay  DelayLength=1  InitialCondition=0
  Delay3 : Delay  InitialCondition=0
  HDL Counter1 : hdlsllib/Sources/HDL Counter  CountType=Count limited  CountInit=0  CountStep=1  CountMax=1  CountFromType=Initial value  CountFrom=0  CountResetPort=off  CountLoadPort=off  CountEnbPort=on  CountDirPort=off  CountHitOutputPort=off  CountDataType=Unsigned  CountWordLen=1  CountFracLen=0  CountSampTime=1
  Logical Operator : Logic  Operator=XOR  AllPortsSameDT=off  OutDataTypeStr=boolean
  Logical Operator1 : Logic  AllPortsSameDT=off  OutDataTypeStr=boolean
  Logical Operator2 : Logic  Operator=NOT  AllPortsSameDT=off  OutDataTypeStr=boolean
  Logical Operator3 : Logic  AllPortsSameDT=off  OutDataTypeStr=boolean
  Logical Operator4 : Logic  AllPortsSameDT=off  OutDataTypeStr=boolean
  Switch : Switch  Criteria=u2 ~= 0  SaturateOnIntegerOverflow=off  InputSameDT=off
  data_out : Outport  VectorParamsAs1DForOutWhenUnconnected=off
  start_out : Outport  Port=2  OutDataTypeStr=boolean  VectorParamsAs1DForOutWhenUnconnected=off
  end_out : Outport  Port=3  OutDataTypeStr=boolean  VectorParamsAs1DForOutWhenUnconnected=off
  valid_out : Outport  Port=4  OutDataTypeStr=boolean  VectorParamsAs1DForOutWhenUnconnected=off
  wires:
  Delay/1 -> Logical Operator/1, Logical Operator1/1, Logical Operator3/1
  Delay3/1 -> data_out/1  "data_out"
  Delay2/1 -> Logical Operator4/2
  Logical Operator/1 -> Switch/3
  Delay1/1 -> Logical Operator/2, Delay2/1  "start_out"
  data_in/1 -> Delay3/1  "data_in"
  end_in/1 -> Delay/1
  Data Type Conversion1/1 -> valid_out/1, Logical Operator3/2, Logical Operator4/1, Logical Operator2/1  "valid_out2"
  HDL Counter1/1 -> Data Type Conversion1/1
  Logical Operator2/1 -> Logical Operator1/2
  Switch/1 -> HDL Counter1/1
  Logical Operator1/1 -> Switch/2
  Constant/1 -> Switch/1
  start_in/1 -> Delay1/1
  Logical Operator4/1 -> start_out/1  "start_out"
  Logical Operator3/1 -> end_out/1  "end_out"

== system tx2/Subsystem6/OFDM_process1/OFDM_process1_bf2/OFDM_BF1/recover_valid_specify ==
  data_in : Inport
  start_in : Inport  Port=2  OutDataTypeStr=boolean
  end_in : Inport  Port=3  OutDataTypeStr=boolean
  Constant : Constant  Value=0  OutDataTypeStr=boolean
  Data Type Conversion1 : DataTypeConversion  OutDataTypeStr=boolean  SaturateOnIntegerOverflow=off  RndMeth=Floor
  Delay : Delay  InitialCondition=0
  Delay1 : Delay  DelayLength=1  InitialCondition=0
  Delay2 : Delay  DelayLength=1  InitialCondition=0
  Delay3 : Delay  InitialCondition=0
  HDL Counter1 : hdlsllib/Sources/HDL Counter  CountType=Count limited  CountInit=0  CountStep=1  CountMax=1  CountFromType=Initial value  CountFrom=0  CountResetPort=off  CountLoadPort=off  CountEnbPort=on  CountDirPort=off  CountHitOutputPort=off  CountDataType=Unsigned  CountWordLen=1  CountFracLen=0  CountSampTime=1
  Logical Operator : Logic  Operator=XOR  AllPortsSameDT=off  OutDataTypeStr=boolean
  Logical Operator1 : Logic  AllPortsSameDT=off  OutDataTypeStr=boolean
  Logical Operator2 : Logic  Operator=NOT  AllPortsSameDT=off  OutDataTypeStr=boolean
  Logical Operator3 : Logic  AllPortsSameDT=off  OutDataTypeStr=boolean
  Logical Operator4 : Logic  AllPortsSameDT=off  OutDataTypeStr=boolean
  Switch : Switch  Criteria=u2 ~= 0  SaturateOnIntegerOverflow=off  InputSameDT=off
  data_out : Outport  VectorParamsAs1DForOutWhenUnconnected=off
  start_out : Outport  Port=2  OutDataTypeStr=boolean  VectorParamsAs1DForOutWhenUnconnected=off
  end_out : Outport  Port=3  OutDataTypeStr=boolean  VectorParamsAs1DForOutWhenUnconnected=off
  valid_out : Outport  Port=4  OutDataTypeStr=boolean  VectorParamsAs1DForOutWhenUnconnected=off
  wires:
  Logical Operator3/1 -> end_out/1  "end_out"
  Logical Operator4/1 -> start_out/1  "start_out"
  start_in/1 -> Delay1/1
  Constant/1 -> Switch/1
  Logical Operator1/1 -> Switch/2
  Switch/1 -> HDL Counter1/1
  Logical Operator2/1 -> Logical Operator1/2
  HDL Counter1/1 -> Data Type Conversion1/1
  Data Type Conversion1/1 -> Logical Operator2/1, Logical Operator4/1, Logical Operator3/2, valid_out/1  "valid_out2"
  end_in/1 -> Delay/1
  data_in/1 -> Delay3/1  "data_in"
  Delay1/1 -> Delay2/1, Logical Operator/2  "start_out"
  Logical Operator/1 -> Switch/3
  Delay2/1 -> Logical Operator4/2
  Delay3/1 -> data_out/1  "data_out"
  Delay/1 -> Logical Operator3/1, Logical Operator1/1, Logical Operator/1

== system tx2/Subsystem6/OFDM_process1/OFDM_process1_bf3/OFDM_BF1/recover_valid_specify ==
  data_in : Inport
  start_in : Inport  Port=2  OutDataTypeStr=boolean
  end_in : Inport  Port=3  OutDataTypeStr=boolean
  Constant : Constant  Value=0  OutDataTypeStr=boolean
  Data Type Conversion1 : DataTypeConversion  OutDataTypeStr=boolean  SaturateOnIntegerOverflow=off  RndMeth=Floor
  Delay : Delay  InitialCondition=0
  Delay1 : Delay  DelayLength=1  InitialCondition=0
  Delay2 : Delay  DelayLength=1  InitialCondition=0
  Delay3 : Delay  InitialCondition=0
  HDL Counter1 : hdlsllib/Sources/HDL Counter  CountType=Count limited  CountInit=0  CountStep=1  CountMax=1  CountFromType=Initial value  CountFrom=0  CountResetPort=off  CountLoadPort=off  CountEnbPort=on  CountDirPort=off  CountHitOutputPort=off  CountDataType=Unsigned  CountWordLen=1  CountFracLen=0  CountSampTime=1
  Logical Operator : Logic  Operator=XOR  AllPortsSameDT=off  OutDataTypeStr=boolean
  Logical Operator1 : Logic  AllPortsSameDT=off  OutDataTypeStr=boolean
  Logical Operator2 : Logic  Operator=NOT  AllPortsSameDT=off  OutDataTypeStr=boolean
  Logical Operator3 : Logic  AllPortsSameDT=off  OutDataTypeStr=boolean
  Logical Operator4 : Logic  AllPortsSameDT=off  OutDataTypeStr=boolean
  Switch : Switch  Criteria=u2 ~= 0  SaturateOnIntegerOverflow=off  InputSameDT=off
  data_out : Outport  VectorParamsAs1DForOutWhenUnconnected=off
  start_out : Outport  Port=2  OutDataTypeStr=boolean  VectorParamsAs1DForOutWhenUnconnected=off
  end_out : Outport  Port=3  OutDataTypeStr=boolean  VectorParamsAs1DForOutWhenUnconnected=off
  valid_out : Outport  Port=4  OutDataTypeStr=boolean  VectorParamsAs1DForOutWhenUnconnected=off
  wires:
  Delay/1 -> Logical Operator/1, Logical Operator1/1, Logical Operator3/1
  Delay3/1 -> data_out/1  "data_out"
  Delay2/1 -> Logical Operator4/2
  Logical Operator/1 -> Switch/3
  Delay1/1 -> Logical Operator/2, Delay2/1  "start_out"
  data_in/1 -> Delay3/1  "data_in"
  end_in/1 -> Delay/1
  Data Type Conversion1/1 -> valid_out/1, Logical Operator3/2, Logical Operator4/1, Logical Operator2/1  "valid_out2"
  HDL Counter1/1 -> Data Type Conversion1/1
  Logical Operator2/1 -> Logical Operator1/2
  Switch/1 -> HDL Counter1/1
  Logical Operator1/1 -> Switch/2
  Constant/1 -> Switch/1
  start_in/1 -> Delay1/1
  Logical Operator4/1 -> start_out/1  "start_out"
  Logical Operator3/1 -> end_out/1  "end_out"

== system tx2/Subsystem6/OFDM_process1/OFDM_process1_bf4/OFDM_BF1/recover_valid_specify ==
  data_in : Inport
  start_in : Inport  Port=2  OutDataTypeStr=boolean
  end_in : Inport  Port=3  OutDataTypeStr=boolean
  Constant : Constant  Value=0  OutDataTypeStr=boolean
  Data Type Conversion1 : DataTypeConversion  OutDataTypeStr=boolean  SaturateOnIntegerOverflow=off  RndMeth=Floor
  Delay : Delay  InitialCondition=0
  Delay1 : Delay  DelayLength=1  InitialCondition=0
  Delay2 : Delay  DelayLength=1  InitialCondition=0
  Delay3 : Delay  InitialCondition=0
  HDL Counter1 : hdlsllib/Sources/HDL Counter  CountType=Count limited  CountInit=0  CountStep=1  CountMax=1  CountFromType=Initial value  CountFrom=0  CountResetPort=off  CountLoadPort=off  CountEnbPort=on  CountDirPort=off  CountHitOutputPort=off  CountDataType=Unsigned  CountWordLen=1  CountFracLen=0  CountSampTime=1
  Logical Operator : Logic  Operator=XOR  AllPortsSameDT=off  OutDataTypeStr=boolean
  Logical Operator1 : Logic  AllPortsSameDT=off  OutDataTypeStr=boolean
  Logical Operator2 : Logic  Operator=NOT  AllPortsSameDT=off  OutDataTypeStr=boolean
  Logical Operator3 : Logic  AllPortsSameDT=off  OutDataTypeStr=boolean
  Logical Operator4 : Logic  AllPortsSameDT=off  OutDataTypeStr=boolean
  Switch : Switch  Criteria=u2 ~= 0  SaturateOnIntegerOverflow=off  InputSameDT=off
  data_out : Outport  VectorParamsAs1DForOutWhenUnconnected=off
  start_out : Outport  Port=2  OutDataTypeStr=boolean  VectorParamsAs1DForOutWhenUnconnected=off
  end_out : Outport  Port=3  OutDataTypeStr=boolean  VectorParamsAs1DForOutWhenUnconnected=off
  valid_out : Outport  Port=4  OutDataTypeStr=boolean  VectorParamsAs1DForOutWhenUnconnected=off
  wires:
  Logical Operator3/1 -> end_out/1  "end_out"
  Logical Operator4/1 -> start_out/1  "start_out"
  start_in/1 -> Delay1/1
  Constant/1 -> Switch/1
  Logical Operator1/1 -> Switch/2
  Switch/1 -> HDL Counter1/1
  Logical Operator2/1 -> Logical Operator1/2
  HDL Counter1/1 -> Data Type Conversion1/1
  Data Type Conversion1/1 -> Logical Operator2/1, Logical Operator4/1, Logical Operator3/2, valid_out/1  "valid_out2"
  end_in/1 -> Delay/1
  data_in/1 -> Delay3/1  "data_in"
  Delay1/1 -> Delay2/1, Logical Operator/2  "start_out"
  Logical Operator/1 -> Switch/3
  Delay2/1 -> Logical Operator4/2
  Delay3/1 -> data_out/1  "data_out"
  Delay/1 -> Logical Operator3/1, Logical Operator1/1, Logical Operator/1
